simulink model "VehicleModel"  (Simulink 10.3)
settings: Solver=ode45  StartTime=0.0  StopTime=tstop  MaxStep=tstep  RelTol=1e-3  EnableMultiTasking=on
InitFcn:
  | addpath(strrep(which(bdroot),[bdroot '.mdl'],''))
  | 
  | InitiateModel;
StopFcn:
  | PlotEVData;
values from neighbouring files (symbols this model uses):
  Av = 2.75    [InitiateModel.m]
  Capacity = 24e3*60*60    (= 86400000)    [InitiateModel.m]
  Cd = 0.29    [InitiateModel.m]
  Cr = 0.01    [InitiateModel.m]
  eta_DC = .98    (= 0.98)    [InitiateModel.m]
  eta_inv = .95    (= 0.95)    [InitiateModel.m]
  Fv_max = Te_max*gratio/rw    (= 5592.34073014)    [InitiateModel.m]
  gratio = 7.94    [InitiateModel.m]
  Ke = 0.407    [InitiateModel.m]
  Kv = 650    [InitiateModel.m]
  Mv = 1620    [InitiateModel.m]
  Pe_max = 80e3    (= 80000)    [InitiateModel.m]
  rho_air = 1.204    [InitiateModel.m]
  rw = 0.4    [InitiateModel.m]
  SOC_0 = 100    [InitiateModel.m]
  Te_max = Pe_max*rw/gratio/Vbase    (= 281.730011594)    [InitiateModel.m]
  Ti = 50    [InitiateModel.m]
  Vbase = 32*0.44704    (= 14.30528)    [InitiateModel.m]
  Vbat = 300    [InitiateModel.m]
  Vbus_ref = 500    [InitiateModel.m]
undefined symbols (not defined in the file or in its folder): MException, motoreff_T, motoreff_w, throw
libraries: simulink x4
settings Model: Creator=ECE  LastModifiedBy=user
settings DataIOCC: LimitDataPoints=on
settings DebuggingCC: SolverPrmCheckMsg=warning  InheritedTsInSrcMsg=none

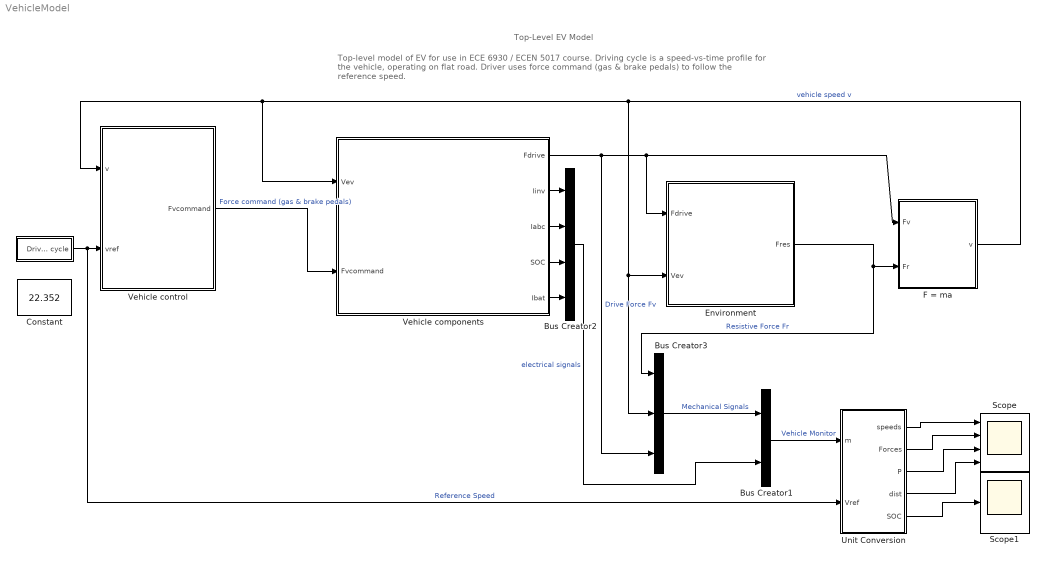
== system VehicleModel ==
  note: Top-level model of EV for use in ECE 6930 / ECEN 5017 course.  Driving cycle is a speed-vs-time
      | profile for the vehicle, operating on flat road.  Driver uses force command (gas & brake
      | pedals) to follow the reference speed.
  note: Top-Level EV Model
  " " : Subsystem  mask{cycle=European (eudc)}
      mask prompts: cycle "Driving cycle"
      mask TypeOptions cycle: US urban (udds) | US highway (hwy) | US supplemental (us06) | European (eudc) | 60 mph constant (mph60)
  Bus Creator1 : BusCreator  Inputs=2
  Bus Creator2 : BusCreator  Inputs=4
  Bus Creator3 : BusCreator  Inputs=3
  Constant : Constant  Value=22.352
  "Environment " : Subsystem
      mask Display:
      | addpath(cd);
      | image(imread('images/road.jpg'))
  F = ma : Subsystem
  Scope : Scope  NumInputPorts=4
  Scope1 : Scope
  Unit Conversion : Subsystem
  Vehicle components : Subsystem
      mask Display:
      | addpath(cd);
      | image(imread('images/EV.png'))
  Vehicle control : Subsystem
      mask Display:
      | addpath(cd);
      | image(imread('images/stig.jpg'))
  wires:
  Vehicle components/1(Fdrive) -> Bus Creator3/3, F = ma/1(Fv), "Environment "/1(Fdrive)  "Drive Force Fv"
  Bus Creator3/1 -> Bus Creator1/1  "Mechanical Signals"
  Bus Creator2/1 -> Bus Creator1/2  "electrical signals"
  Vehicle components/2(Iinv) -> Bus Creator2/1
  Vehicle components/3(Iabc) -> Bus Creator2/2
  Vehicle components/4(SOC) -> Bus Creator2/3
  Vehicle components/5(Ibat) -> Bus Creator2/4
  Unit Conversion/1(speeds) -> Scope/1
  Unit Conversion/2(Forces) -> Scope/2
  Unit Conversion/3(P) -> Scope/3
  Unit Conversion/4(dist) -> Scope/4
  Unit Conversion/5(SOC) -> Scope1/1
  Vehicle control/1(Fvcommand) -> Vehicle components/2(Fvcommand)  "Force command (gas & brake pedals)"
  "Environment "/1(Fres) -> F = ma/2(Fr), Bus Creator3/1  "Resistive Force Fr"
  F = ma/1(v) -> Vehicle control/1(v), Vehicle components/1(Vev), "Environment "/2(Vev), Bus Creator3/2  "vehicle speed v"
  Bus Creator1/1 -> Unit Conversion/1(m)  "Vehicle Monitor"
  " "/1(Driving cycle) -> Unit Conversion/2(Vref), Vehicle control/2(vref)  "Reference Speed"

== system VehicleModel/  ==
  Constant : Constant  Value=cycle
  Multiport Switch : MultiPortSwitch  Inputs=5  SaturateOnIntegerOverflow=on  InputSameDT=on
  v-buss1 : FromWorkspace  VariableName=us06  SampleTime=-1  ZeroCross=off  OutputAfterFinalValue=Setting to zero
  v-buss2 : FromWorkspace  VariableName=udds  SampleTime=-1  ZeroCross=off  OutputAfterFinalValue=Setting to zero
  v-buss3 : FromWorkspace  VariableName=hwy  SampleTime=-1  ZeroCross=off  OutputAfterFinalValue=Setting to zero
  v-buss4 : FromWorkspace  VariableName=mph60  SampleTime=-1  ZeroCross=off  OutputAfterFinalValue=Setting to zero
  v-buss8 : FromWorkspace  VariableName=eudc  SampleTime=-1  ZeroCross=off  OutputAfterFinalValue=Setting to zero
  Driving cycle : Outport
  wires:
  Constant/1 -> Multiport Switch/1
  Multiport Switch/1 -> Driving cycle/1
  v-buss8/1 -> Multiport Switch/5
  v-buss2/1 -> Multiport Switch/2
  v-buss3/1 -> Multiport Switch/3
  v-buss1/1 -> Multiport Switch/4
  v-buss4/1 -> Multiport Switch/6

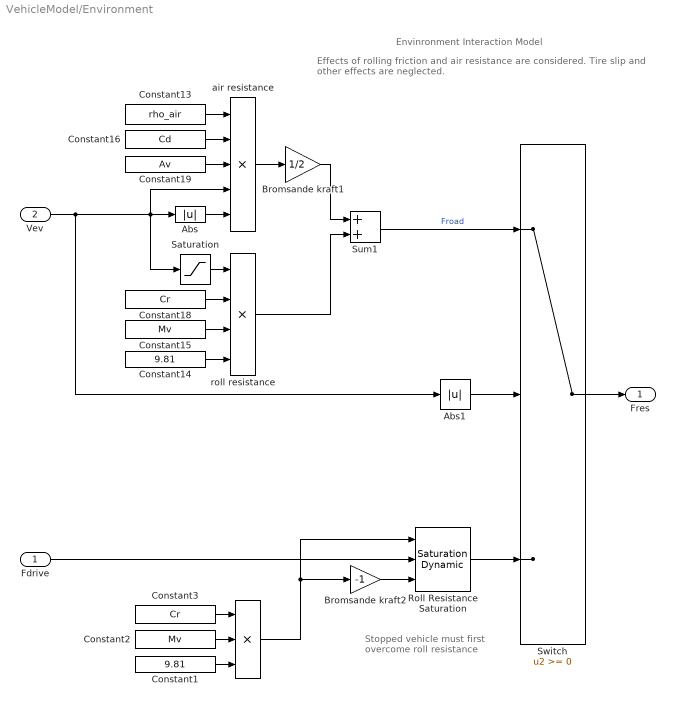
== system VehicleModel/Environment  ==
  note: Stopped vehicle must first
      | overcome roll resistance
  note: Effects of rolling friction and air resistance are considered.  Tire slip
      | and other effects are neglected.
  note: Envinronment Interaction Model
  Fdrive : Inport
  Vev : Inport  Port=2
  "   " : Product  Inputs=3  InputSameDT=on  SaturateOnIntegerOverflow=on  OutDataTypeStr=Inherit: Same as first input
  Abs : Abs  SaturateOnIntegerOverflow=on
  Abs1 : Abs
  Bromsande kraft1 : Gain  Gain=1/2  SaturateOnIntegerOverflow=on  OutDataTypeStr=Inherit: Same as input  ParamDataTypeStr=Inherit: Same as input
  Bromsande kraft2 : Gain  Gain=-1  SaturateOnIntegerOverflow=on  OutDataTypeStr=Inherit: Same as input  ParamDataTypeStr=Inherit: Same as input
  Constant1 : Constant  Value=9.81
  Constant13 : Constant  Value=rho_air
  Constant14 : Constant  Value=9.81
  Constant15 : Constant  Value=Mv
  Constant16 : Constant  Value=Cd
  Constant18 : Constant  Value=Cr
  Constant19 : Constant  Value=Av
  Constant2 : Constant  Value=Mv
  Constant3 : Constant  Value=Cr
  Roll Resistance Saturation : simulink/Discontinuities/Saturation Dynamic  OutMin=[]  OutMax=[]  OutDataTypeStr=Inherit: Same as second input  OutDataType=fixdt(1, 16)  OutScaling=2^-10  DoSatur=off
  Saturation : Saturate  UpperLimit=1  LowerLimit=-1
  Sum1 : Sum  InputSameDT=on  SaturateOnIntegerOverflow=on  OutDataTypeStr=Inherit: Same as first input
  Switch : Switch
  air resistance : Product  Inputs=5  InputSameDT=on  SaturateOnIntegerOverflow=on  OutDataTypeStr=Inherit: Same as first input
  roll resistance : Product  Inputs=4  InputSameDT=on  SaturateOnIntegerOverflow=on  OutDataTypeStr=Inherit: Same as first input
  Fres : Outport  InitialOutput=0
  wires:
  air resistance/1 -> Bromsande kraft1/1
  Bromsande kraft1/1 -> Sum1/1
  Constant13/1 -> air resistance/1
  Constant16/1 -> air resistance/2
  Constant19/1 -> air resistance/3
  Constant18/1 -> roll resistance/2
  Constant15/1 -> roll resistance/3
  Constant14/1 -> roll resistance/4
  Abs/1 -> air resistance/5
  Saturation/1 -> roll resistance/1
  Sum1/1 -> Switch/1  "Froad"
  Vev/1 -> Abs1/1, air resistance/4, Saturation/1, Abs/1
  roll resistance/1 -> Sum1/2
  Switch/1 -> Fres/1
  Roll Resistance Saturation/1 -> Switch/3
  Abs1/1 -> Switch/2
  Fdrive/1 -> Roll Resistance Saturation/2
  Constant3/1 -> "   "/1
  Constant2/1 -> "   "/2
  Constant1/1 -> "   "/3
  "   "/1 -> Roll Resistance Saturation/1, Bromsande kraft2/1
  Bromsande kraft2/1 -> Roll Resistance Saturation/3

== system VehicleModel/F = ma ==
  Fv : Inport
  Fr : Inport  Port=2
  "   " : Sum  Inputs=+-
  Acceleration [m/s^2] to speed [m/s] : Integrator
  Force [N] to  acceleration [m/s^2] : Gain  Gain=1/Mv
  v : Outport
  wires:
  "   "/1 -> Force [N] to  acceleration [m/s^2]/1  "Net Force"
  Force [N] to  acceleration [m/s^2]/1 -> Acceleration [m/s^2] to speed [m/s]/1  "Vehicle Acceleration"
  Fv/1 -> "   "/1
  Fr/1 -> "   "/2
  Acceleration [m/s^2] to speed [m/s]/1 -> v/1  "Vehicle Speed"

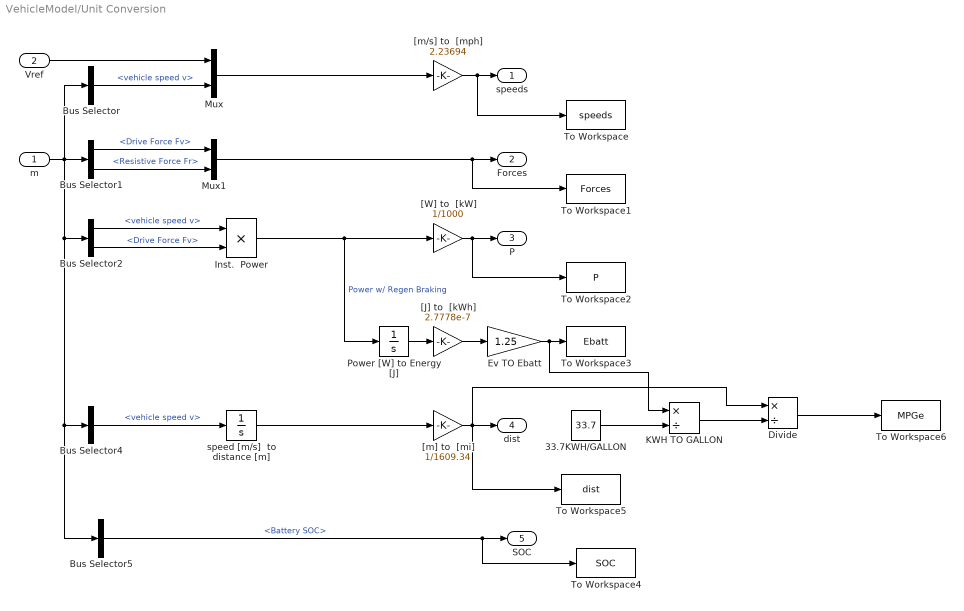
== system VehicleModel/Unit Conversion ==
  m : Inport
  Vref : Inport  Port=2
  33.7KWH/GALLON : Constant  Value=33.7
  Bus Selector : BusSelector  OutputSignals=Mechanical Signals.vehicle speed v
  Bus Selector1 : BusSelector  OutputSignals=Mechanical Signals.Drive Force Fv,Mechanical Signals.Resistive Force Fr
  Bus Selector2 : BusSelector  OutputSignals=Mechanical Signals.vehicle speed v,Mechanical Signals.Drive Force Fv
  Bus Selector4 : BusSelector  OutputSignals=Mechanical Signals.vehicle speed v
  Bus Selector5 : BusSelector  OutputSignals=electrical signals.Battery SOC
  Divide : Product  Inputs=*/
  Ev TO Ebatt : Gain  Gain=1.25
  Inst.  Power : Product  RndMeth=Zero
  KWH TO GALLON : Product  Inputs=*/
  Mux : Mux  Inputs=2
  Mux1 : Mux  Inputs=2
  Power [W] to Energy [J] : Integrator
  To Workspace : ToWorkspace  VariableName=speeds  SaveFormat=Structure With Time  SampleTime=-1
  To Workspace1 : ToWorkspace  VariableName=Forces  SaveFormat=Structure With Time  SampleTime=-1
  To Workspace2 : ToWorkspace  VariableName=P  SaveFormat=Structure With Time  SampleTime=-1
  To Workspace3 : ToWorkspace  VariableName=Ebatt  SaveFormat=Structure With Time  SampleTime=-1
  To Workspace4 : ToWorkspace  VariableName=SOC  SaveFormat=Structure With Time  SampleTime=-1
  To Workspace5 : ToWorkspace  VariableName=dist  SaveFormat=Structure With Time  SampleTime=-1
  To Workspace6 : ToWorkspace  VariableName=MPGe  SaveFormat=Structure With Time  SampleTime=-1
  "[J] to  [kWh]" : Gain  Gain=2.7778e-7
  "[W] to  [kW]" : Gain  Gain=1/1000
  "[m/s] to  [mph]" : Gain  Gain=2.23694
  "[m] to  [mi]" : Gain  Gain=1/1609.34
  speed [m/s]  to distance [m] : Integrator
  speeds : Outport
  Forces : Outport  Port=2
  P : Outport  Port=3
  dist : Outport  Port=4
  SOC : Outport  Port=5
  wires:
  Mux/1 -> "[m/s] to  [mph]"/1
  "[m/s] to  [mph]"/1 -> speeds/1, To Workspace/1
  Mux1/1 -> Forces/1, To Workspace1/1
  Bus Selector2/1 -> Inst.  Power/1  "<vehicle speed v>"
  Bus Selector4/1 -> speed [m/s]  to distance [m]/1  "<vehicle speed v>"
  speed [m/s]  to distance [m]/1 -> "[m] to  [mi]"/1
  "[m] to  [mi]"/1 -> Divide/1, dist/1, To Workspace5/1
  Bus Selector/1 -> Mux/2  "<vehicle speed v>"
  Vref/1 -> Mux/1
  Bus Selector1/1 -> Mux1/1  "<Drive Force Fv>"
  Bus Selector1/2 -> Mux1/2  "<Resistive Force Fr>"
  Bus Selector2/2 -> Inst.  Power/2  "<Drive Force Fv>"
  "[W] to  [kW]"/1 -> P/1, To Workspace2/1
  Power [W] to Energy [J]/1 -> "[J] to  [kWh]"/1
  "[J] to  [kWh]"/1 -> Ev TO Ebatt/1
  Inst.  Power/1 -> "[W] to  [kW]"/1, Power [W] to Energy [J]/1  "Power w/ Regen Braking"
  Bus Selector5/1 -> SOC/1, To Workspace4/1  "<Battery SOC>"
  m/1 -> Bus Selector/1, Bus Selector1/1, Bus Selector2/1, Bus Selector4/1, Bus Selector5/1
  Ev TO Ebatt/1 -> KWH TO GALLON/1, To Workspace3/1
  Divide/1 -> To Workspace6/1
  KWH TO GALLON/1 -> Divide/2
  33.7KWH/GALLON/1 -> KWH TO GALLON/2

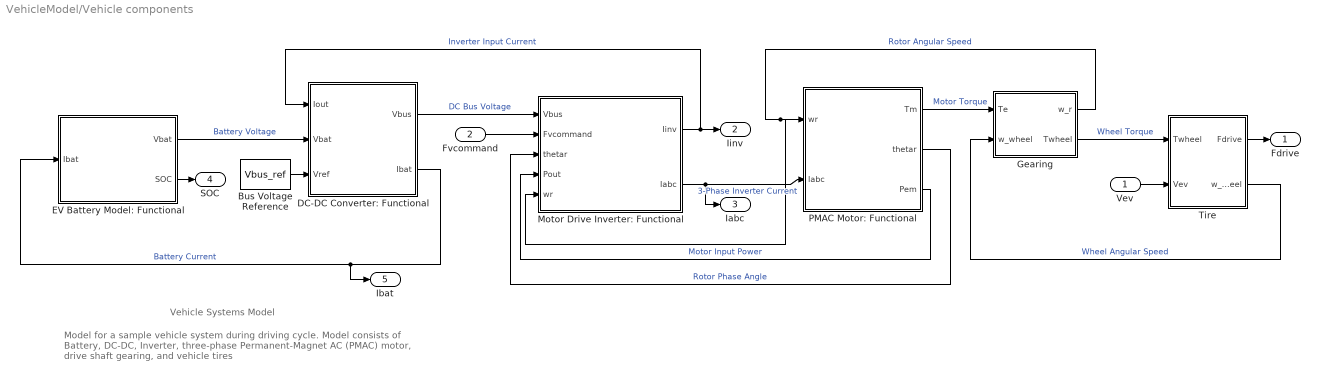
== system VehicleModel/Vehicle components ==
  note: Vehicle Systems Model
  note: Model for a sample vehicle system during driving cycle.  Model consists
      | of Battery, DC-DC, Inverter, three-phase Permanent-Magnet AC
      | (PMAC) motor, drive shaft gearing, and vehicle tires
  Vev : Inport
  Fvcommand : Inport  Port=2
  Bus Voltage Reference : Constant  Value=Vbus_ref
  DC-DC Converter: Functional : Subsystem
      mask Display:
      | addpath(cd);
      | image(imread('images/DC-DC.jpg'))
  EV Battery Model: Functional : Subsystem
      mask Display:
      | addpath(cd);
      | image(imread('images/battery.jpg'))
  Gearing : Subsystem
      mask Display:
      | addpath(cd);
      | image(imread('images/Transmission.png'))
  Motor Drive Inverter: Functional : Subsystem
      mask Display:
      | addpath(cd);
      | image(imread('images/inverter.jpg'))
  PMAC Motor: Functional : Subsystem
      mask Display:
      | addpath(cd);
      | image(imread('images/motor.jpg'))
  Tire : Subsystem
      mask Display:
      | addpath(cd);
      | image(imread('images/tire.jpg'))
  Fdrive : Outport
  Iinv : Outport  Port=2
  Iabc : Outport  Port=3
  SOC : Outport  Port=4
  Ibat : Outport  Port=5
  wires:
  EV Battery Model: Functional/1(Vbat) -> DC-DC Converter: Functional/2(Vbat)  "Battery Voltage"
  DC-DC Converter: Functional/2(Ibat) -> EV Battery Model: Functional/1(Ibat), Ibat/1  "Battery Current"
  EV Battery Model: Functional/2(SOC) -> SOC/1
  Motor Drive Inverter: Functional/2(Iabc) -> PMAC Motor: Functional/2(Iabc), Iabc/1  "3-Phase Inverter Current"
  Bus Voltage Reference/1 -> DC-DC Converter: Functional/3(Vref)
  PMAC Motor: Functional/2(thetar) -> Motor Drive Inverter: Functional/3(thetar)  "Rotor Phase Angle"
  Motor Drive Inverter: Functional/1(Iinv) -> DC-DC Converter: Functional/1(Iout), Iinv/1  "Inverter Input Current"
  DC-DC Converter: Functional/1(Vbus) -> Motor Drive Inverter: Functional/1(Vbus)  "DC Bus Voltage"
  PMAC Motor: Functional/3(Pem) -> Motor Drive Inverter: Functional/4(Pout)  "Motor Input Power"
  Tire/1(Fdrive) -> Fdrive/1
  Vev/1 -> Tire/2(Vev)
  PMAC Motor: Functional/1(Tm) -> Gearing/1(Te)  "Motor Torque"
  Gearing/2(Twheel) -> Tire/1(Twheel)  "Wheel Torque"
  Tire/2(w_wheel) -> Gearing/2(w_wheel)  "Wheel Angular Speed"
  Gearing/1(w_r) -> PMAC Motor: Functional/1(wr), Motor Drive Inverter: Functional/5(wr)  "Rotor Angular Speed"
  Fvcommand/1 -> Motor Drive Inverter: Functional/2(Fvcommand)

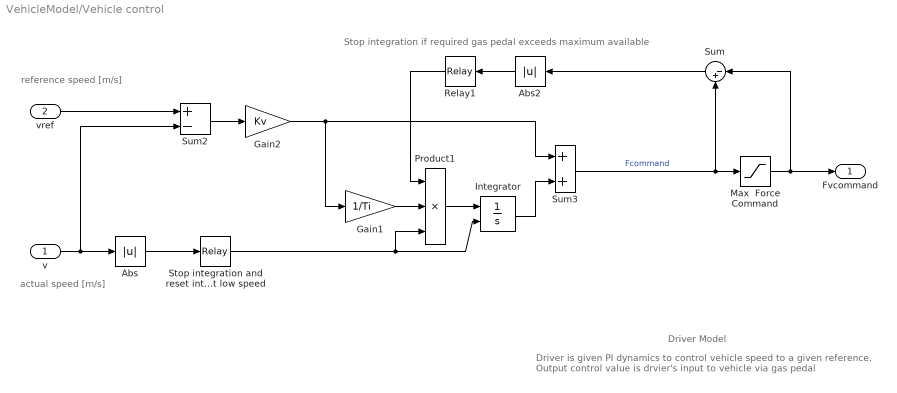
== system VehicleModel/Vehicle control ==
  note: Stop integration if required gas pedal exceeds maximum available
  note: actual
      | speed [m/s]
  note: reference
      | speed [m/s]
  note: Driver is given PI dynamics to control vehicle speed to a given reference.
      | Output control value is drvier's input to vehicle via gas pedal
  note: Driver Model
  v : Inport
  vref : Inport  Port=2
  Abs : Abs  SaturateOnIntegerOverflow=on
  Abs2 : Abs  SaturateOnIntegerOverflow=on
  Gain1 : Gain  Gain=1/Ti  SaturateOnIntegerOverflow=on  OutDataTypeStr=Inherit: Same as input  ParamDataTypeStr=Inherit: Same as input
  Gain2 : Gain  Gain=Kv  SaturateOnIntegerOverflow=on  OutDataTypeStr=Inherit: Same as input  ParamDataTypeStr=Inherit: Same as input
  Integrator : Integrator  ExternalReset=falling  UpperSaturationLimit=1000  LowerSaturationLimit=-10000
  Max  Force Command : Saturate  UpperLimit=Fv_max  LowerLimit=-Fv_max
  Product1 : Product  Inputs=3  InputSameDT=on  SaturateOnIntegerOverflow=on  OutDataTypeStr=Inherit: Same as first input
  Relay1 : Relay  OnOutputValue=0  OffOutputValue=1
  Stop integration and reset integrator at low speed : Relay  OnSwitchValue=0.3  OffSwitchValue=0.3-eps
  Sum : Sum  Inputs=|-+
  Sum2 : Sum  Inputs=+-  InputSameDT=on  SaturateOnIntegerOverflow=on  OutDataTypeStr=Inherit: Same as first input
  Sum3 : Sum  InputSameDT=on  SaturateOnIntegerOverflow=on  OutDataTypeStr=Inherit: Same as first input
  Fvcommand : Outport  InitialOutput=0
  wires:
  Relay1/1 -> Product1/1
  Abs2/1 -> Relay1/1
  Sum/1 -> Abs2/1
  Max  Force Command/1 -> Sum/1, Fvcommand/1
  Gain1/1 -> Product1/2
  Abs/1 -> Stop integration and reset integrator at low speed/1
  Product1/1 -> Integrator/1
  Sum3/1 -> Sum/2, Max  Force Command/1  "Fcommand"
  Integrator/1 -> Sum3/2
  Gain2/1 -> Gain1/1, Sum3/1
  Stop integration and reset integrator at low speed/1 -> Product1/3, Integrator/2
  Sum2/1 -> Gain2/1
  vref/1 -> Sum2/1
  v/1 -> Abs/1, Sum2/2

== system VehicleModel/Vehicle components/DC-DC Converter: Functional ==
  note: DC-DC converter consists of power stage
      | model and controller, which drives the bus
      | voltage to a given reference by varying
      | converter duty cycle
  note: DC-DC Functional Model
  Iout : Inport
  Vbat : Inport  Port=2
  Vref : Inport  Port=3
  DC/DC Controller1 : Subsystem
  "DC/DC Model:  Functional " : Subsystem
  Vbus : Outport
  Ibat : Outport  Port=2
  wires:
  "DC/DC Model:  Functional "/1(Vout) -> DC/DC Controller1/1(Vbus), Vbus/1
  DC/DC Controller1/1(D) -> "DC/DC Model:  Functional "/3(D)
  Vref/1 -> DC/DC Controller1/2(Vref)
  Iout/1 -> "DC/DC Model:  Functional "/1(Iout)
  Vbat/1 -> "DC/DC Model:  Functional "/2(Vbat)
  "DC/DC Model:  Functional "/2(Ibat) -> Ibat/1

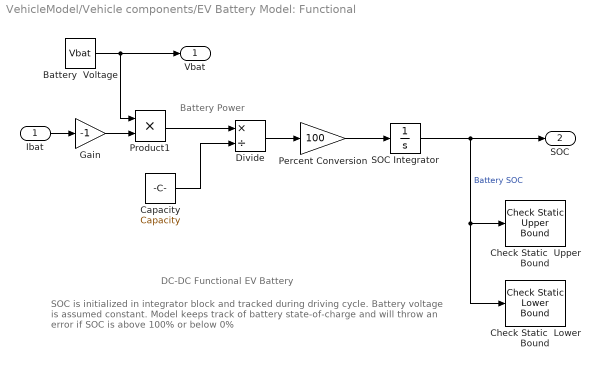
== system VehicleModel/Vehicle components/EV Battery Model: Functional ==
  note: Battery
      | Power
  note: SOC is initialized in integrator block and tracked during driving cycle.  Battery
      | voltage is assumed constant.  Model keeps track of battery state-of-charge and
      | will throw an error if SOC is above 100% or below 0%
  note: DC-DC Functional EV Battery
  Ibat : Inport
  Battery  Voltage : Constant  Value=Vbat
  Capacity : Constant  Value=Capacity
  Check Static  Lower Bound : simulink/Model Verification/Check Static  Lower Bound  Description=0-eps <= u  min=0-eps  min_included=on  enabled=on  callback=throw(MException('ResultChk:OutOfRange','Battery SOC has fallen below 0'))  stopWhenAssertionFail=on  export=off  icon=graphic
  Check Static  Upper Bound : simulink/Model Verification/Check Static  Upper Bound  Description=u <= 100+eps  max=100+eps  max_included=on  enabled=on  callback=throw(MException('ResultChk:OutOfRange','Battery SOC has exceeded 100'))  stopWhenAssertionFail=on  export=off  icon=graphic
      settings: SourceProductBaseCode=SL
  Divide : Product  Inputs=*/
  Gain : Gain  Gain=-1
  Percent Conversion : Gain  Gain=100
  Product1 : Product  RndMeth=Zero
  SOC Integrator : Integrator  InitialCondition=SOC_0
  Vbat : Outport
  SOC : Outport  Port=2
  wires:
  Ibat/1 -> Gain/1
  Product1/1 -> Divide/1
  SOC Integrator/1 -> SOC/1, Check Static  Upper Bound/1, Check Static  Lower Bound/1  "Battery SOC"
  Battery  Voltage/1 -> Vbat/1, Product1/1
  Gain/1 -> Product1/2
  Capacity/1 -> Divide/2
  Divide/1 -> Percent Conversion/1
  Percent Conversion/1 -> SOC Integrator/1

== system VehicleModel/Vehicle components/Gearing ==
  note: Model of connection between motor and wheel.  In this
      | example, it is assumed that motor and wheel are directly coupled
      | by an ideal, lossless shaft with no gear reduction.
  note: Vehicle Transmission Model
  Te : Inport
  w_wheel : Inport  Port=2
  Constant : Constant  Value=gratio
  Product : Product  RndMeth=Zero
  Product1 : Product  RndMeth=Zero
  w_r : Outport
  Twheel : Outport  Port=2
  wires:
  Te/1 -> Product/1
  w_wheel/1 -> Product1/2
  Product/1 -> Twheel/1
  Product1/1 -> w_r/1
  Constant/1 -> Product/2, Product1/1

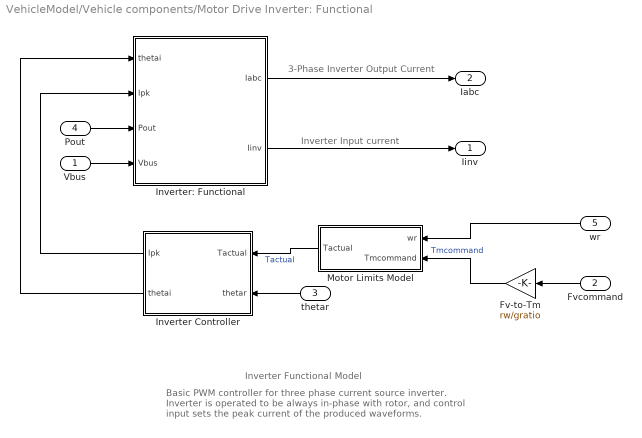
== system VehicleModel/Vehicle components/Motor Drive Inverter: Functional ==
  note: 3-Phase Inverter Output Current
  note: Inverter Input current
  note: Basic PWM controller for three phase current source inverter.
      | Inverter is operated to be always in-phase with rotor,
      | and control input sets the peak current of the produced
      | waveforms.
  note: Inverter Functional Model
  Vbus : Inport
  Fvcommand : Inport  Port=2
  thetar : Inport  Port=3
  Pout : Inport  Port=4
  wr : Inport  Port=5
  Fv-to-Tm : Gain  Gain=rw/gratio
  Inverter Controller : Subsystem
  Inverter: Functional : Subsystem
  Motor Limits Model : Subsystem
  Iinv : Outport
  Iabc : Outport  Port=2
  wires:
  Inverter Controller/2(thetai) -> Inverter: Functional/1(thetai)
  Inverter Controller/1(Ipk) -> Inverter: Functional/2(Ipk)
  Inverter: Functional/2(Iinv) -> Iinv/1
  Inverter: Functional/1(Iabc) -> Iabc/1
  thetar/1 -> Inverter Controller/2(thetar)
  Pout/1 -> Inverter: Functional/3(Pout)
  Vbus/1 -> Inverter: Functional/4(Vbus)
  Motor Limits Model/1(Tactual) -> Inverter Controller/1(Tactual)  "Tactual"
  wr/1 -> Motor Limits Model/1(wr)
  Fvcommand/1 -> Fv-to-Tm/1
  Fv-to-Tm/1 -> Motor Limits Model/2(Tmcommand)  "Tmcommand"

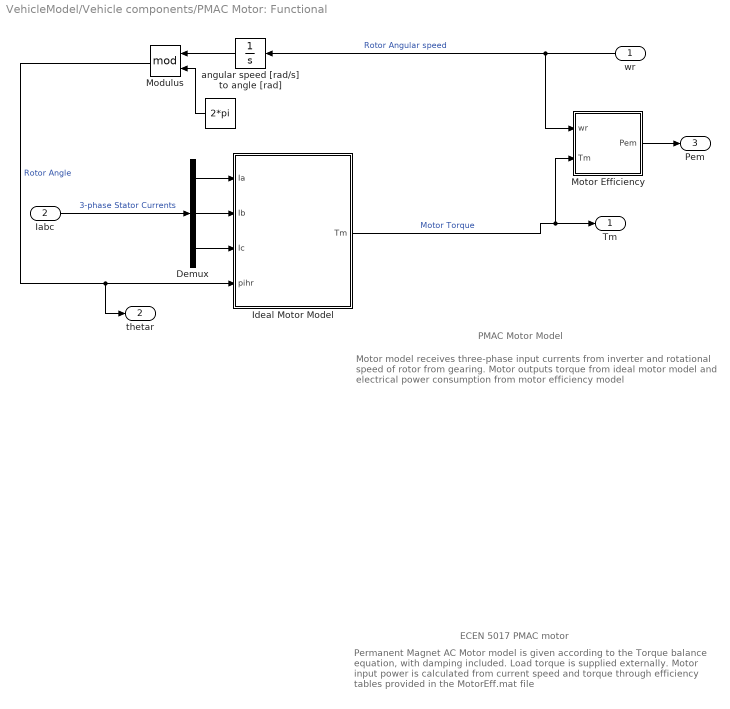
== system VehicleModel/Vehicle components/PMAC Motor: Functional ==
  note: Permanent Magnet AC Motor model is given according to the
      | Torque balance equation, with damping included.  Load torque is supplied
      | externally.  Motor input power is calculated from current speed and torque
      | through efficiency tables provided in the MotorEff.mat file
  note: ECEN 5017 PMAC motor
  note: PMAC Motor Model
  note: Motor model receives three-phase input currents from inverter and
      | rotational speed of rotor from gearing.  Motor outputs torque from ideal
      | motor model and electrical power consumption from motor efficiency model
  wr : Inport
  Iabc : Inport  Port=2
  " " : Constant  Value=2*pi
  Demux : Demux  Outputs=3
  Ideal Motor Model : Subsystem
  Modulus : Math  Operator=mod  SignedPower=on  SaturateOnIntegerOverflow=on
  Motor Efficiency : Subsystem
  angular speed [rad/s] to angle [rad] : Integrator
  Tm : Outport
  thetar : Outport  Port=2
  Pem : Outport  Port=3
  wires:
  wr/1 -> Motor Efficiency/1(wr), angular speed [rad/s] to angle [rad]/1  "Rotor Angular speed"
  Iabc/1 -> Demux/1  "3-phase Stator Currents"
  Motor Efficiency/1(Pem) -> Pem/1
  Demux/3 -> Ideal Motor Model/3(Ic)
  Demux/2 -> Ideal Motor Model/2(Ib)
  Demux/1 -> Ideal Motor Model/1(Ia)
  Modulus/1 -> Ideal Motor Model/4(pihr), thetar/1  "Rotor Angle"
  angular speed [rad/s] to angle [rad]/1 -> Modulus/1
  Ideal Motor Model/1(Tm) -> Tm/1, Motor Efficiency/2(Tm)  "Motor Torque"
  " "/1 -> Modulus/2

== system VehicleModel/Vehicle components/Tire ==
  note: Model of tire used to convert from rotational to linear mechanics.
      | Slip and other higher order effects are not considered.
  note: Vehicle Tire Model
  Twheel : Inport
  Vev : Inport  Port=2
  Linear Speed [m/s] to Angular [rad/s] : Gain  Gain=1/rw
  torque [Nm] to  Force [N] : Gain  Gain=1/rw
  Fdrive : Outport
  w_wheel : Outport  Port=2
  wires:
  torque [Nm] to  Force [N]/1 -> Fdrive/1
  Vev/1 -> Linear Speed [m/s] to Angular [rad/s]/1
  Linear Speed [m/s] to Angular [rad/s]/1 -> w_wheel/1
  Twheel/1 -> torque [Nm] to  Force [N]/1

== system VehicleModel/Vehicle components/DC-DC Converter: Functional/DC/DC Controller1 ==
  note: Basic PWM controller for DC-DC Boost converter.
      | Compensator is pure integral to ensure zero
      | steady-state error.  No dynamics considered. Duty
      | cycle is limited between 0 and 1
  note: DC-DC Functional Controller
  Vbus : Inport
  Vref : Inport  Port=2
  Gain : Gain
  Integrator : Integrator  InitialCondition=.5
  Saturation : Saturate  UpperLimit=1  LowerLimit=0
  Sum : Sum  Inputs=|-+
  D : Outport
  wires:
  Gain/1 -> Integrator/1
  Integrator/1 -> Saturation/1
  Sum/1 -> Gain/1
  Vbus/1 -> Sum/1
  Vref/1 -> Sum/2
  Saturation/1 -> D/1

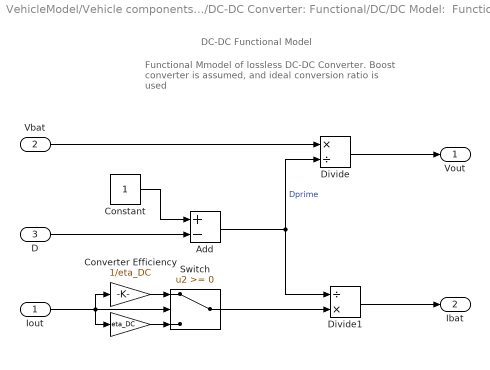
== system VehicleModel/Vehicle components/DC-DC Converter: Functional/DC/DC Model:  Functional  ==
  note: Functional Mmodel of lossless DC-DC Converter.
      | Boost converter is assumed, and ideal conversion
      | ratio is used
  note: DC-DC Functional Model
  Iout : Inport
  Vbat : Inport  Port=2
  D : Inport  Port=3
  "  " : Gain  Gain=eta_DC
  Add : Sum  Inputs=+-
  Constant : Constant
  Converter Efficiency : Gain  Gain=1/eta_DC
  Divide : Product  Inputs=*/
  Divide1 : Product  Inputs=/*
  Switch : Switch
  Vout : Outport
  Ibat : Outport  Port=2
  wires:
  Constant/1 -> Add/1
  D/1 -> Add/2
  Add/1 -> Divide/2, Divide1/1  "Dprime"
  Vbat/1 -> Divide/1
  Divide/1 -> Vout/1
  Iout/1 -> Switch/2, Converter Efficiency/1, "  "/1
  Divide1/1 -> Ibat/1
  Switch/1 -> Divide1/2
  Converter Efficiency/1 -> Switch/1
  "  "/1 -> Switch/3

== system VehicleModel/Vehicle components/Motor Drive Inverter: Functional/Inverter Controller ==
  note: Inverter is kept in phase with rotor, and torque command is used
      | to directly set peak currents, which ultimately determine engine torque.
      | Because ideal sensing/control are assumed, no dynamics are considered
  note: Inverter Functional Controller
  Tactual : Inport
  thetar : Inport  Port=2
  Torque [Nm] to  Inverter Peak Current [A] : Gain  Gain=1/Ke*2/3
  Ipk : Outport
  thetai : Outport  Port=2
  wires:
  thetar/1 -> thetai/1
  Torque [Nm] to  Inverter Peak Current [A]/1 -> Ipk/1
  Tactual/1 -> Torque [Nm] to  Inverter Peak Current [A]/1

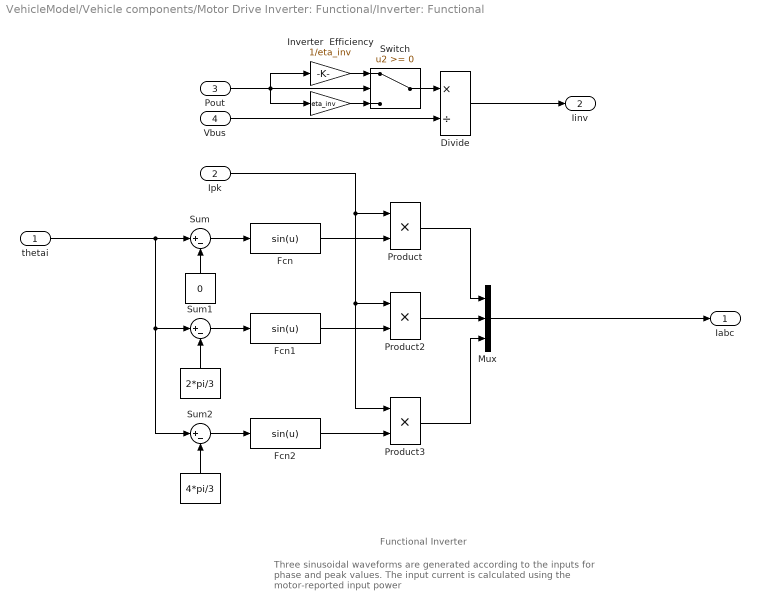
== system VehicleModel/Vehicle components/Motor Drive Inverter: Functional/Inverter: Functional ==
  note: Three sinusoidal waveforms are generated according to the inputs
      | for phase and peak values.  The input current is calculated using
      | the motor-reported input power
  note: Functional Inverter
  thetai : Inport
  Ipk : Inport  Port=2
  Pout : Inport  Port=3
  Vbus : Inport  Port=4
  "  " : Gain  Gain=eta_inv
  " " : Constant  Value=0
  "   " : Constant  Value=2*pi/3
  "    " : Constant  Value=4*pi/3
  " Fcn" : Fcn  Expr=sin(u)
  Divide : Product  Inputs=*/
  Fcn1 : Fcn  Expr=sin(u)
  Fcn2 : Fcn  Expr=sin(u)
  Inverter  Efficiency : Gain  Gain=1/eta_inv
  Mux : Mux  Inputs=3
  Product : Product  RndMeth=Zero
  Product2 : Product  RndMeth=Zero
  Product3 : Product  RndMeth=Zero
  Sum : Sum  Inputs=|+-
  Sum1 : Sum  Inputs=|+-
  Sum2 : Sum  Inputs=|+-
  Switch : Switch
  Iabc : Outport
  Iinv : Outport  Port=2
  wires:
  " Fcn"/1 -> Product/2
  Product/1 -> Mux/1
  Ipk/1 -> Product/1, Product2/1, Product3/1
  Sum/1 -> " Fcn"/1
  Fcn1/1 -> Product2/2
  Sum1/1 -> Fcn1/1
  Fcn2/1 -> Product3/2
  Sum2/1 -> Fcn2/1
  Product2/1 -> Mux/2
  Product3/1 -> Mux/3
  " "/1 -> Sum/2
  "   "/1 -> Sum1/2
  "    "/1 -> Sum2/2
  thetai/1 -> Sum/1, Sum1/1, Sum2/1
  Mux/1 -> Iabc/1
  Pout/1 -> Switch/2, Inverter  Efficiency/1, "  "/1
  Vbus/1 -> Divide/2
  Divide/1 -> Iinv/1
  Switch/1 -> Divide/1
  Inverter  Efficiency/1 -> Switch/1
  "  "/1 -> Switch/3

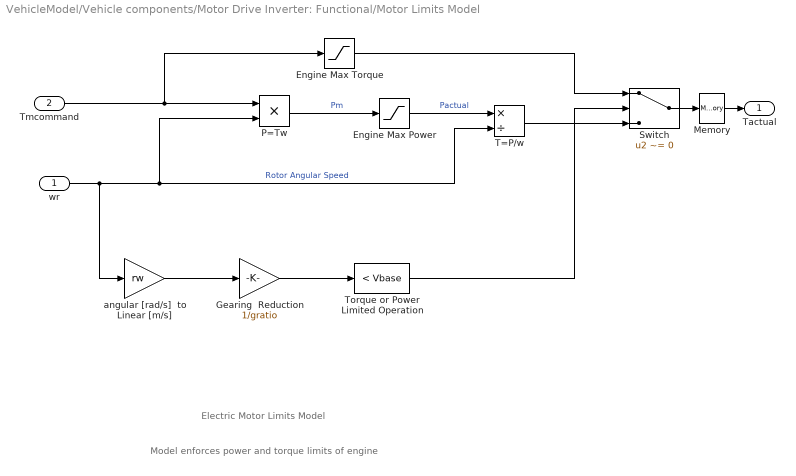
== system VehicleModel/Vehicle components/Motor Drive Inverter: Functional/Motor Limits Model ==
  note: Electric Motor Limits Model
  note: Model enforces power and torque limits of engine
  wr : Inport
  Tmcommand : Inport  Port=2
  Engine Max Power : Saturate  UpperLimit=Pe_max  LowerLimit=-Pe_max
  Engine Max Torque : Saturate  UpperLimit=Te_max  LowerLimit=-Te_max
  Gearing  Reduction : Gain  Gain=1/gratio
  Memory : Memory
  P=Tw : Product  RndMeth=Zero
  Switch : Switch  Criteria=u2 ~= 0
  T=P/w : Product  Inputs=*/
  Torque or Power Limited Operation : simulink/Logic and Bit Operations/Compare To Constant  relop=<  const=Vbase  OutDataTypeStr=uint8  ZeroCross=off
  angular [rad/s]  to Linear [m/s] : Gain  Gain=rw
  Tactual : Outport
  wires:
  Tmcommand/1 -> P=Tw/1, Engine Max Torque/1
  P=Tw/1 -> Engine Max Power/1  "Pm"
  Engine Max Power/1 -> T=P/w/1  "Pactual"
  Switch/1 -> Memory/1
  T=P/w/1 -> Switch/3
  Torque or Power Limited Operation/1 -> Switch/2
  Engine Max Torque/1 -> Switch/1
  Memory/1 -> Tactual/1
  angular [rad/s]  to Linear [m/s]/1 -> Gearing  Reduction/1
  wr/1 -> P=Tw/2, T=P/w/2, angular [rad/s]  to Linear [m/s]/1  "Rotor Angular Speed"
  Gearing  Reduction/1 -> Torque or Power Limited Operation/1

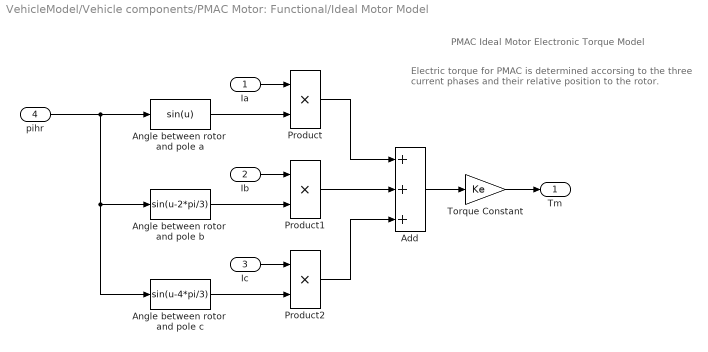
== system VehicleModel/Vehicle components/PMAC Motor: Functional/Ideal Motor Model ==
  note: Electric torque for PMAC is determined accorsing to the three
      | current phases and their relative position to the rotor.
  note: PMAC Ideal Motor Electronic Torque Model
  Ia : Inport
  Ib : Inport  Port=2
  Ic : Inport  Port=3
  pihr : Inport  Port=4
  Add : Sum  Inputs=+++
  Angle between rotor  and pole a : Fcn  Expr=sin(u)
  Angle between rotor  and pole b : Fcn  Expr=sin(u-2*pi/3)
  Angle between rotor  and pole c : Fcn  Expr=sin(u-4*pi/3)
  Product : Product  RndMeth=Zero
  Product1 : Product  RndMeth=Zero
  Product2 : Product  RndMeth=Zero
  Torque Constant : Gain  Gain=Ke
  Tm : Outport
  wires:
  pihr/1 -> Angle between rotor  and pole a/1, Angle between rotor  and pole b/1, Angle between rotor  and pole c/1
  Angle between rotor  and pole a/1 -> Product/2
  Ia/1 -> Product/1
  Ib/1 -> Product1/1
  Angle between rotor  and pole b/1 -> Product1/2
  Ic/1 -> Product2/1
  Angle between rotor  and pole c/1 -> Product2/2
  Add/1 -> Torque Constant/1
  Product/1 -> Add/1
  Product1/1 -> Add/2
  Product2/1 -> Add/3
  Torque Constant/1 -> Tm/1

== system VehicleModel/Vehicle components/PMAC Motor: Functional/Motor Efficiency ==
  note: PMAC Motor Efficiency Model
  note: Angular speed and torque are used to compute mechanical power.  Then, speed
      | and torque are used as indices into a 2-d lookup table for motor efficiency
  wr : Inport
  Tm : Inport  Port=2
  2-D Lookup Table : Lookup_n-D  BreakpointsForDimension1=motoreff_w  BreakpointsForDimension2=motoreff_T  Table=motoreff'  ExtrapMethod=Clip  UseLastTableValue=on  RndMeth=Simplest  InputSameDT=on
      settings: InputPortMap=u0,u1
  Abs : Abs
  Abs1 : Abs
  Divide : Product  Inputs=*/
  Math Function : Math  Operator=reciprocal  SignedPower=on  SaturateOnIntegerOverflow=on
  Product : Product  RndMeth=Zero
  Saturation : Saturate  UpperLimit=1  LowerLimit=.05
  Switch : Switch
  Pem : Outport
  wires:
  Divide/1 -> Pem/1
  Abs/1 -> 2-D Lookup Table/2
  Abs1/1 -> 2-D Lookup Table/1
  2-D Lookup Table/1 -> Saturation/1
  wr/1 -> Abs1/1, Product/1
  Tm/1 -> Abs/1, Product/2
  Switch/1 -> Divide/2
  Product/1 -> Divide/1, Switch/2
  Saturation/1 -> Math Function/1, Switch/1
  Math Function/1 -> Switch/3
